simulink model "DC_Motor"  (R2024b)
settings: Solver=VariableStepAuto  StartTime=0.0  StopTime=30  RelTol=1e-3
settings Model: Creator=marvincalmer  LastModifiedBy=marvincalmer
settings HardwareCC: ProdBitPerPointer=32  ProdBitPerSizeT=32  ProdBitPerPtrDiffT=32  ProdWordSize=32  ProdHWDeviceType=Intel->x86-32 (Windows32)

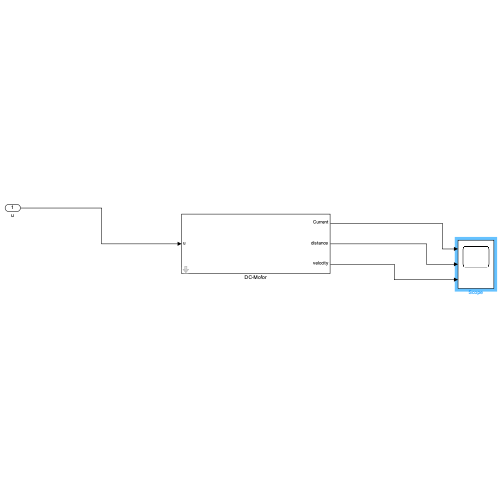
[thumbnail: Simulink's stored preview of the top-level diagram]
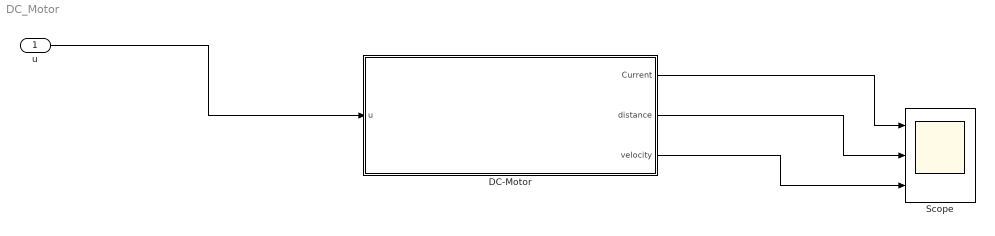
== system DC_Motor ==
  u : Inport
  DC-Motor : Subsystem  mask{R=0.083, L=0.000087, k_M=0.161, m=0.1, d=0.09, i0=10, x0=1, x_dot0=1}
      mask prompts: i0 "Starting current"; x0 "Starting distance"; x_dot0 "Starting current"
  Scope : Scope  NumInputPorts=3
  wires:
  u/1 -> DC-Motor/1(u)
  DC-Motor/3(velocity) -> Scope/3
  DC-Motor/2(distance) -> Scope/2
  DC-Motor/1(Current) -> Scope/1

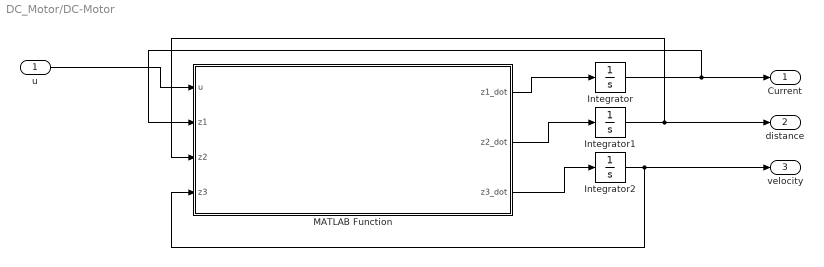
== system DC_Motor/DC-Motor ==
  u : Inport
  Integrator : Integrator  InitialCondition=i0
  Integrator1 : Integrator  InitialCondition=x0
  Integrator2 : Integrator  InitialCondition=x_dot0
  MATLAB Function : MATLAB Function  TreatAsAtomicUnit=on
  Current : Outport
  distance : Outport  Port=2
  velocity : Outport  Port=3
  wires:
  u/1 -> MATLAB Function/1(u)
  MATLAB Function/2(z2_dot) -> Integrator1/1
  Integrator1/1 -> MATLAB Function/3(z2), distance/1
  MATLAB Function/3(z3_dot) -> Integrator2/1
  MATLAB Function/1(z1_dot) -> Integrator/1
  Integrator/1 -> MATLAB Function/2(z1), Current/1
  Integrator2/1 -> MATLAB Function/4(z3), velocity/1

== matlab function DC_Motor/DC-Motor/MATLAB Function ==
  data: u input; z1_dot output; z1 input; z2 input; z3 input; z2_dot output; z3_dot output; k_M parameter; L parameter; R parameter; m parameter; d parameter
function [z1_dot,z2_dot,z3_dot] = fcn(u,z1,z2,z3,k_M, L, R, m, d)
    %params
    % R=1;
    % L=1e-3;
    % k_M=1;
    % m=1;
    % d=1;

    %DGL
    z1_dot = -(R/L)*z1-(k_M/L)*z2+(1/L)*u;
    z2_dot = z3;
    z3_dot = (k_M/m)*z1-(d/m)*z3;

    

end
